simulink model "Assignment_1"  (R2022a)
settings: Solver=FixedStepAuto  StartTime=0.0  StopTime=1  FixedStep=1e-3  RelTol=1e-3  EnableMultiTasking=on
undefined symbols (not defined in the file or in its folder): D0, D1, D10, D11, D12, D13, D2, D3, D4, D5, D6, D7, D8, D9, PTA0, PTA1, PTA2, PTB23, PTB9, PTC16, PTC17, PTC2, PTC3, PTC4, PTD0, PTD1, PTD2, PTD3
libraries: frdmk64flib x14
settings Model: ExtModeTrigDuration=5  Creator=anand  LastModifiedBy=anand
settings OptimizationCC: EnhancedBackFolding=on  PassReuseOutputArgsAs=Individual arguments  ZeroExternalMemoryAtStartup=off  ZeroInternalMemoryAtStartup=off  MaxStackSize=64  OptimizeBlockOrder=speed  DifferentSizesBufferReuse=on  OptimizationCustomize=off  EfficientTunableParamExpr=on
settings DebuggingCC: ParameterTunabilityLossMsg=error
settings HardwareCC: ProdBitPerPointer=32  ProdBitPerSizeT=32  ProdBitPerPtrDiffT=32  ProdLargestAtomicInteger=Long  ProdLargestAtomicFloat=Double  ProdWordSize=32  ProdHWDeviceType=ARM Compatible->ARM Cortex
settings SFSimCC: MATLABDynamicMemAlloc=off
settings RTWCC: SystemTargetFile=ert.tlc  HardwareBoard=NXP FRDM-K64F  TLCOptions="-aInlineSetEventsForThisBaseRateFcn=TLC_FALSE -aSuppressMultiTaskScheduler=TLC_FALSE  -aRateBasedStepFcn=0"  TemplateMakefile=ert_default_tmf  Toolchain=GNU Tools for ARM Embedded Processors
settings CodeAppCC: ForceParamTrailComments=on  IgnoreCustomStorageClasses=off  OperatorAnnotations=on  SimulinkDataObjDesc=on  SFDataObjDesc=on  InsertBlockDesc=on
settings ERTTargetCC: ExtModeTransport=4  ExtModeMexFile=sendToCommService

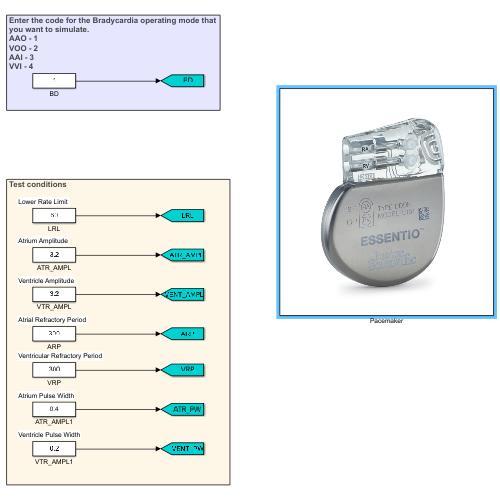
[thumbnail: Simulink's stored preview of the top-level diagram]
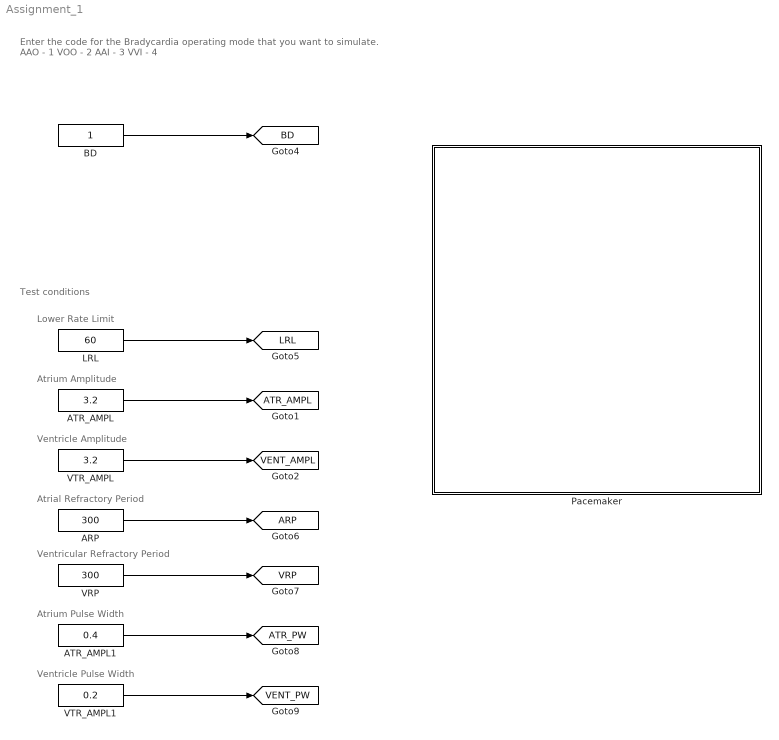
== system Assignment_1 ==
  note: Lower Rate Limit
  note: Test conditions
  note: Enter the code for the Bradycardia operating mode that
      | you want to simulate.
      | AAO - 1
      | VOO - 2
      | AAI - 3
      | VVI - 4
  note: Atrium Amplitude
  note: Ventricle Amplitude
  note: Atrial Refractory Period
  note: Ventricular Refractory Period
  note: Atrium Pulse Width
  note: Ventricle Pulse Width
  ARP : Constant  Value=300
  ATR_AMPL : Constant  Value=3.2
  ATR_AMPL1 : Constant  Value=0.4
  BD : Constant
  LRL : Constant  Value=60
  Pacemaker : Subsystem
      mask Display: image('$imagefile'); % Use "Edit Image" on toolstrip to change.
  VRP : Constant  Value=300
  VTR_AMPL : Constant  Value=3.2
  VTR_AMPL1 : Constant  Value=0.2
  tag scope: ARP=global, ATR_AMPL=global, ATR_PW=global, BD=global, LRL=global, VENT_AMPL=global, VENT_PW=global, VRP=global
  wires:
  LRL/1 -> [LRL]
  BD/1 -> [BD]
  ATR_AMPL/1 -> [ATR_AMPL]
  VTR_AMPL/1 -> [VENT_AMPL]
  ARP/1 -> [ARP]
  VRP/1 -> [VRP]
  ATR_AMPL1/1 -> [ATR_PW]
  VTR_AMPL1/1 -> [VENT_PW]

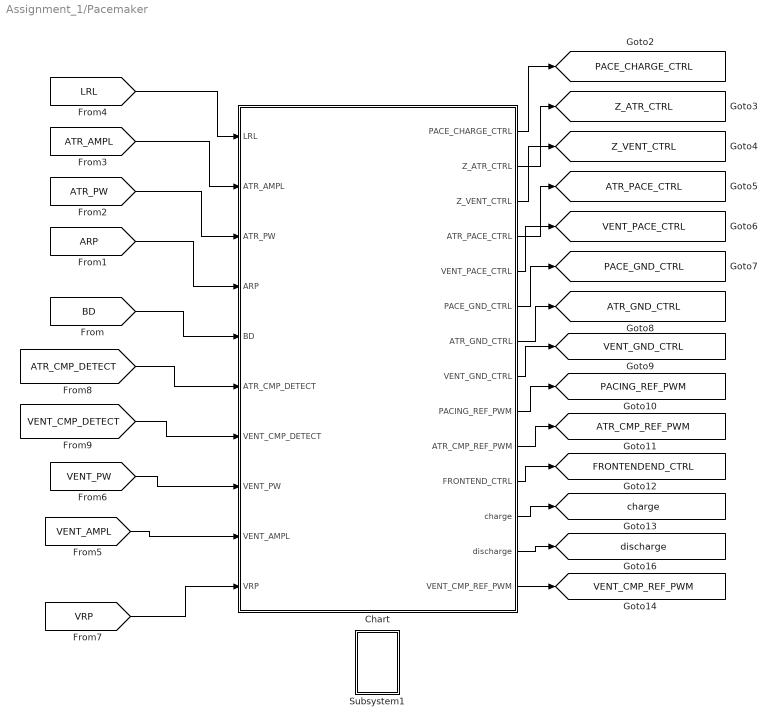
== system Assignment_1/Pacemaker ==
  Chart : Stateflow chart  TreatAsAtomicUnit=on
  Subsystem1 : Subsystem
  tag scope: ATR_CMP_REF_PWM=global, ATR_GND_CTRL=global, ATR_PACE_CTRL=global, FRONTENDEND_CTRL=global, PACE_CHARGE_CTRL=global, PACE_GND_CTRL=global, PACING_REF_PWM=global, VENT_CMP_REF_PWM=global, VENT_GND_CTRL=global, VENT_PACE_CTRL=global, Z_ATR_CTRL=global, Z_VENT_CTRL=global, charge=global, discharge=global
  wires:
  [BD] -> Chart/5(BD)
  [ATR_AMPL] -> Chart/2(ATR_AMPL)
  [ARP] -> Chart/4(ARP)
  [LRL] -> Chart/1(LRL)
  [ATR_PW] -> Chart/3(ATR_PW)
  [VENT_AMPL] -> Chart/9(VENT_AMPL)
  [VENT_PW] -> Chart/8(VENT_PW)
  [VRP] -> Chart/10(VRP)
  [ATR_CMP_DETECT] -> Chart/6(ATR_CMP_DETECT)
  [VENT_CMP_DETECT] -> Chart/7(VENT_CMP_DETECT)
  Chart/1(PACE_CHARGE_CTRL) -> [PACE_CHARGE_CTRL]
  Chart/2(Z_ATR_CTRL) -> [Z_ATR_CTRL]
  Chart/3(Z_VENT_CTRL) -> [Z_VENT_CTRL]
  Chart/11(FRONTEND_CTRL) -> [FRONTENDEND_CTRL]
  Chart/10(ATR_CMP_REF_PWM) -> [ATR_CMP_REF_PWM]
  Chart/9(PACING_REF_PWM) -> [PACING_REF_PWM]
  Chart/4(ATR_PACE_CTRL) -> [ATR_PACE_CTRL]
  Chart/5(VENT_PACE_CTRL) -> [VENT_PACE_CTRL]
  Chart/6(PACE_GND_CTRL) -> [PACE_GND_CTRL]
  Chart/7(ATR_GND_CTRL) -> [ATR_GND_CTRL]
  Chart/8(VENT_GND_CTRL) -> [VENT_GND_CTRL]
  Chart/12(charge) -> [charge]
  Chart/13(discharge) -> [discharge]
  Chart/14(VENT_CMP_REF_PWM) -> [VENT_CMP_REF_PWM]

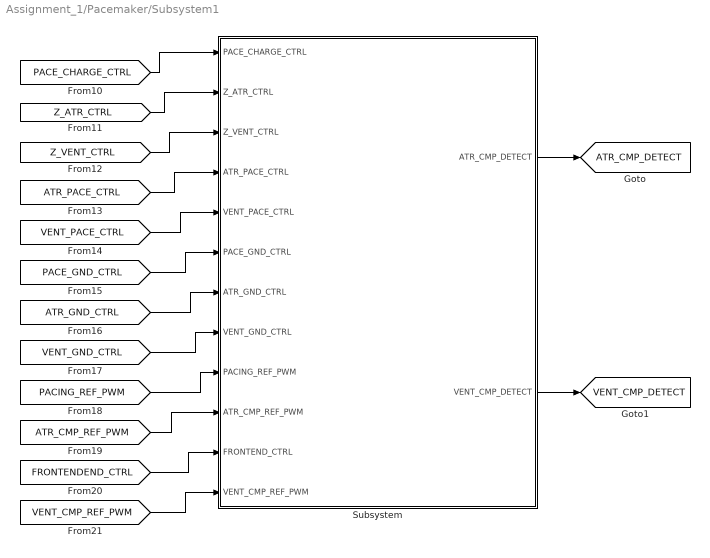
== system Assignment_1/Pacemaker/Subsystem1 ==
  Subsystem : Subsystem
  tag scope: ATR_CMP_DETECT=global, VENT_CMP_DETECT=global
  wires:
  [PACE_GND_CTRL] -> Subsystem/6(PACE_GND_CTRL)
  Subsystem/1(ATR_CMP_DETECT) -> [ATR_CMP_DETECT]
  [Z_ATR_CTRL] -> Subsystem/2(Z_ATR_CTRL)
  [FRONTENDEND_CTRL] -> Subsystem/11(FRONTEND_CTRL)
  [ATR_CMP_REF_PWM] -> Subsystem/10(ATR_CMP_REF_PWM)
  [Z_VENT_CTRL] -> Subsystem/3(Z_VENT_CTRL)
  Subsystem/2(VENT_CMP_DETECT) -> [VENT_CMP_DETECT]
  [PACE_CHARGE_CTRL] -> Subsystem/1(PACE_CHARGE_CTRL)
  [VENT_GND_CTRL] -> Subsystem/8(VENT_GND_CTRL)
  [ATR_GND_CTRL] -> Subsystem/7(ATR_GND_CTRL)
  [PACING_REF_PWM] -> Subsystem/9(PACING_REF_PWM)
  [VENT_PACE_CTRL] -> Subsystem/5(VENT_PACE_CTRL)
  [ATR_PACE_CTRL] -> Subsystem/4(ATR_PACE_CTRL)
  [VENT_CMP_REF_PWM] -> Subsystem/12(VENT_CMP_REF_PWM)

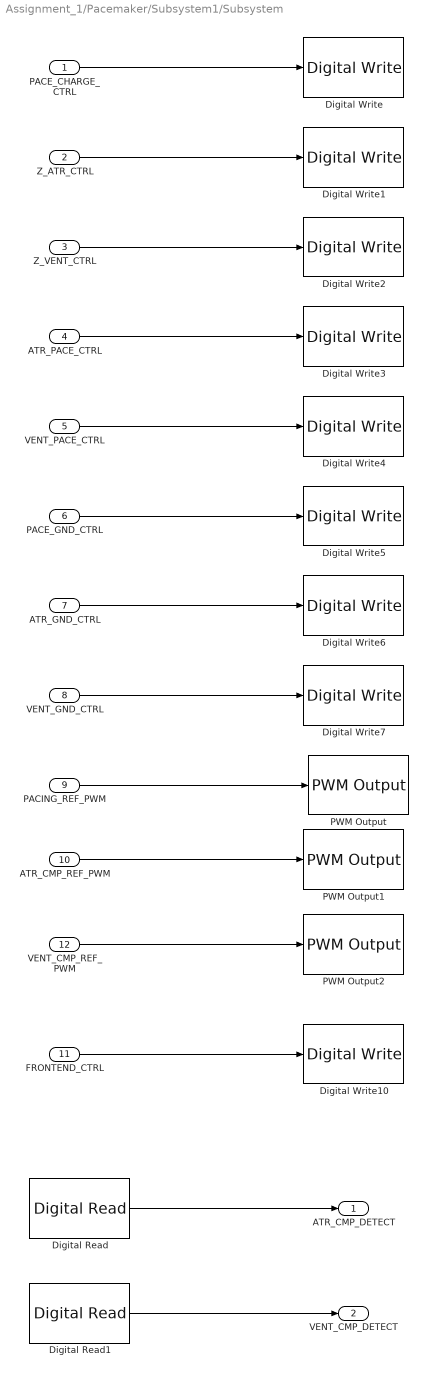
== system Assignment_1/Pacemaker/Subsystem1/Subsystem ==
  PACE_CHARGE_CTRL : Inport  OutDataTypeStr=boolean
  Z_ATR_CTRL : Inport  Port=2  OutDataTypeStr=boolean
  Z_VENT_CTRL : Inport  Port=3
  ATR_PACE_CTRL : Inport  Port=4
  VENT_PACE_CTRL : Inport  Port=5
  PACE_GND_CTRL : Inport  Port=6
  ATR_GND_CTRL : Inport  Port=7
  VENT_GND_CTRL : Inport  Port=8
  PACING_REF_PWM : Inport  Port=9
  ATR_CMP_REF_PWM : Inport  Port=10
  FRONTEND_CTRL : Inport  Port=11
  VENT_CMP_REF_PWM : Inport  Port=12
  Digital Read : frdmk64flib/Digital Read  Whichpin=PTC16 (D0)  SampleTime=-1
  Digital Read1 : frdmk64flib/Digital Read  Whichpin=PTC17 (D1)  SampleTime=-1
  Digital Write : frdmk64flib/Digital Write  Whichpin=PTB9 (D2)
  Digital Write1 : frdmk64flib/Digital Write  Whichpin=PTB23 (D4)
  Digital Write10 : frdmk64flib/Digital Write  Whichpin=PTD1 (D13)
  Digital Write2 : frdmk64flib/Digital Write  Whichpin=PTC3 (D7)
  Digital Write3 : frdmk64flib/Digital Write  Whichpin=PTA0 (D8)
  Digital Write4 : frdmk64flib/Digital Write  Whichpin=PTC4 (D9)
  Digital Write5 : frdmk64flib/Digital Write  Whichpin=PTD0 (D10)
  Digital Write6 : frdmk64flib/Digital Write  Whichpin=PTD2 (D11)
  Digital Write7 : frdmk64flib/Digital Write  Whichpin=PTD3 (D12)
  PWM Output : frdmk64flib/PWM Output  Whichpin=PTA2 (D5)  InitialFrequency=2000  InitialDutyCycle=0
  PWM Output1 : frdmk64flib/PWM Output  Whichpin=PTC2 (D6)  InitialFrequency=2000  InitialDutyCycle=0
  PWM Output2 : frdmk64flib/PWM Output  Whichpin=PTA1 (D3)  InitialFrequency=2000  InitialDutyCycle=0
  ATR_CMP_DETECT : Outport  OutDataTypeStr=boolean
  VENT_CMP_DETECT : Outport  Port=2  OutDataTypeStr=boolean
  wires:
  PACE_CHARGE_CTRL/1 -> Digital Write/1
  Z_ATR_CTRL/1 -> Digital Write1/1
  Z_VENT_CTRL/1 -> Digital Write2/1
  ATR_PACE_CTRL/1 -> Digital Write3/1
  VENT_PACE_CTRL/1 -> Digital Write4/1
  PACE_GND_CTRL/1 -> Digital Write5/1
  ATR_GND_CTRL/1 -> Digital Write6/1
  VENT_GND_CTRL/1 -> Digital Write7/1
  PACING_REF_PWM/1 -> PWM Output/1
  ATR_CMP_REF_PWM/1 -> PWM Output1/1
  Digital Read/1 -> ATR_CMP_DETECT/1
  FRONTEND_CTRL/1 -> Digital Write10/1
  Digital Read1/1 -> VENT_CMP_DETECT/1
  VENT_CMP_REF_PWM/1 -> PWM Output2/1

== stateflow chart Assignment_1/Pacemaker/Chart ==
  state AOO
    state CHARGING_DISCHARGING
      entry:
      charge = true;
      %DISCHARGING C21
      PACE_GND_CTRL = true;
      VENT_PACE_CTRL = false;
      Z_ATR_CTRL = false;
      Z_VENT_CTRL = false;
      ATR_PACE_CTRL = false;
      ATR_GND_CTRL = true;
      VENT_GND_CTRL = false;
      %CHARGING C22
      PACING_REF_PWM = 100*ATR_AMPL/5;
      PACE_CHARGE_CTRL = true;
    state PACE_ATR
      entry:
      charge = false;
      PACE_CHARGE_CTRL = false;
      PACE_GND_CTRL = true;
      ATR_PACE_CTRL = true;
      ATR_GND_CTRL = false;
      Z_ATR_CTRL = false;
      Z_VENT_CTRL = false;
      VENT_GND_CTRL = false;
      VENT_PACE_CTRL = false;
    (default) -> AOO.CHARGING_DISCHARGING
    AOO.CHARGING_DISCHARGING -> AOO.PACE_ATR : [after(60000/LRL-ATR_PW, msec)]
    AOO.PACE_ATR -> AOO.CHARGING_DISCHARGING : [after(ATR_PW,msec)]
  state VOO
    state CHARGING_DISCHARGING
      entry:
      charge = true;
      %DISCHARGING C21
      PACE_GND_CTRL = true;
      VENT_PACE_CTRL = false;
      Z_ATR_CTRL = false;
      Z_VENT_CTRL = false;
      ATR_PACE_CTRL = false;
      ATR_GND_CTRL = true;
      VENT_GND_CTRL = false;
      %CHARGING C22
      PACING_REF_PWM = 100*VENT_AMPL/5;
      PACE_CHARGE_CTRL = true;
    state PACE_ATR
      entry:
      charge = false;
      PACE_CHARGE_CTRL = false;
      PACE_GND_CTRL = true;
      ATR_PACE_CTRL = false;
      ATR_GND_CTRL = false;
      Z_ATR_CTRL = false;
      Z_VENT_CTRL = false;
      VENT_GND_CTRL = false;
      VENT_PACE_CTRL = true;
    (default) -> VOO.CHARGING_DISCHARGING
    VOO.CHARGING_DISCHARGING -> VOO.PACE_ATR : [after(60000/LRL-VENT_PW, msec)]
    VOO.PACE_ATR -> VOO.CHARGING_DISCHARGING : [after(VENT_PW,msec)]
  state Start
    entry:
  state AAI
    state CHARGING
      entry:
      %CHARGING C22
      charge = true;
      discharge = false;
      FRONTEND_CTRL = true;
      VENT_PACE_CTRL = false;
      ATR_PACE_CTRL = false;
      PACE_CHARGE_CTRL = true;
      PACING_REF_PWM = 90;
      ATR_CMP_REF_PWM = 75;
    state PACE_ATR
      entry:
      charge = false;
      discharge = false;
      PACE_CHARGE_CTRL = false;
      PACE_GND_CTRL = true;
      VENT_PACE_CTRL = false;
      VENT_GND_CTRL = false;
      Z_VENT_CTRL = false;
      Z_ATR_CTRL = false;
      ATR_GND_CTRL = false;
      ATR_PACE_CTRL = true;
    state Atrial_Refractory_Period_Post_Sensing
      entry:
    state DISCHARGING
      entry:
      %DISCHARGING C21
      charge = false;
      discharge = true;
      PACE_GND_CTRL = true;
      ATR_PACE_CTRL = false;
      Z_VENT_CTRL = false;
      Z_ATR_CTRL = false;
      VENT_PACE_CTRL = false;
      VENT_GND_CTRL = false;
      ATR_GND_CTRL = true;
    (default) -> AAI.CHARGING : {delta = 0; sensing = 0}
    AAI.CHARGING -> Atrial_Refractory_Period_Post_Sensing [order 1] : [ATR_CMP_DETECT == true]
    AAI.CHARGING -> AAI.PACE_ATR [order 2] : [after(60000/LRL-delta-ATR_PW, msec)]
    Atrial_Refractory_Period_Post_Sensing -> AAI.CHARGING : [after(ARP+10,msec)]{delta = ARP; sensing = 1}
    (junction 210) -> AAI.CHARGING : [after(1, msec)]{delta = 0; sensing = 0}
    (junction 198) -> AAI.CHARGING : [after(ARP,msec)]{delta = ARP}
    AAI.PACE_ATR -> AAI.DISCHARGING : [after(ATR_PW,msec)]
    AAI.DISCHARGING -> (junction 198) [order 1] : [sensing == 0]
    AAI.DISCHARGING -> (junction 210) [order 2] : [sensing == 1]
  state VVI
    state CHARGING
      entry:
      %CHARGING C22
      FRONTEND_CTRL = true;
      ATR_PACE_CTRL = false;
      VENT_PACE_CTRL = false;
      PACING_REF_PWM = 90;
      PACE_CHARGE_CTRL = true;
      VENT_CMP_REF_PWM = 75;
    state PACE_ATR
      entry:
      PACE_CHARGE_CTRL = false;
      PACE_GND_CTRL = true;
      ATR_PACE_CTRL = false;
      ATR_GND_CTRL = false;
      Z_ATR_CTRL = false;
      Z_VENT_CTRL = false;
      VENT_GND_CTRL = false;
      VENT_PACE_CTRL = true;
    state Ventricular_Refractory_Period_Post_Sensing
      entry:
    state DISCHARGING
      entry:
      %DISCHARGING C21
      PACE_GND_CTRL = true;
      VENT_PACE_CTRL = false;
      Z_ATR_CTRL = false;
      Z_VENT_CTRL = false;
      ATR_PACE_CTRL = false;
      ATR_GND_CTRL = false;
      VENT_GND_CTRL = true;
    (default) -> VVI.CHARGING : {delta = 0; sensing = 0}
    VVI.CHARGING -> Ventricular_Refractory_Period_Post_Sensing [order 1] : [VENT_CMP_DETECT == true]
    VVI.CHARGING -> VVI.PACE_ATR [order 2] : [after(60000/LRL-delta-VENT_PW, msec)]
    Ventricular_Refractory_Period_Post_Sensing -> VVI.CHARGING : [after(VRP+30,msec)]{delta = VRP; sensing = 1}
    (junction 215) -> VVI.CHARGING : [after(1, msec)]{delta = 0; sensing = 0}
    (junction 214) -> VVI.CHARGING : [after(VRP,msec)]{delta = VRP}
    VVI.PACE_ATR -> VVI.DISCHARGING : [after(VENT_PW,msec)]
    VVI.DISCHARGING -> (junction 214) [order 1] : [sensing == 0]
    VVI.DISCHARGING -> (junction 215) [order 2] : [sensing == 1]
  Start -> AOO [order 1] : [BD == 1]
  Start -> VOO [order 2] : [BD == 2]
  (default) -> Start
  Start -> AAI [order 3] : [BD == 3]
  Start -> VVI [order 4] : [BD == 4]
  data: LRL input size=[1]; ATR_AMPL input size=[1]; ATR_PW input size=[1]; PACE_CHARGE_CTRL output boolean; Z_ATR_CTRL output; Z_VENT_CTRL output; ATR_PACE_CTRL output; VENT_PACE_CTRL output; PACE_GND_CTRL output; ATR_GND_CTRL output; VENT_GND_CTRL output; PACING_REF_PWM output; ARP input size=[1]; ATR_CMP_REF_PWM output; delta local double; FRONTEND_CTRL output; BD input size=[1]; ATR_CMP_DETECT input boolean size=[1,1]; VENT_CMP_DETECT input boolean size=[1,1]; sensing local; VENT_PW input size=[1]; VENT_AMPL input size=[1]; charge output boolean; discharge output boolean; VENT_CMP_REF_PWM output; VRP input
